simulink model "MesurementModel"  (R2023b)
settings: configuration reference "Configuration" (kept outside this file)
libraries: dspstat3 x4, SignalEditorBlockLib x1
settings Model: DataDictionary=ZC_EVPowerSystem.sldd  Creator=ykamatan  LastModifiedBy=ykamatan
settings ConfigSetRef: SourceName=Configuration

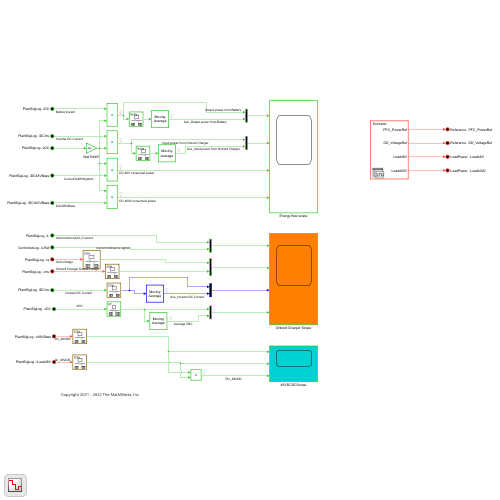
[thumbnail: Simulink's stored preview of the top-level diagram]
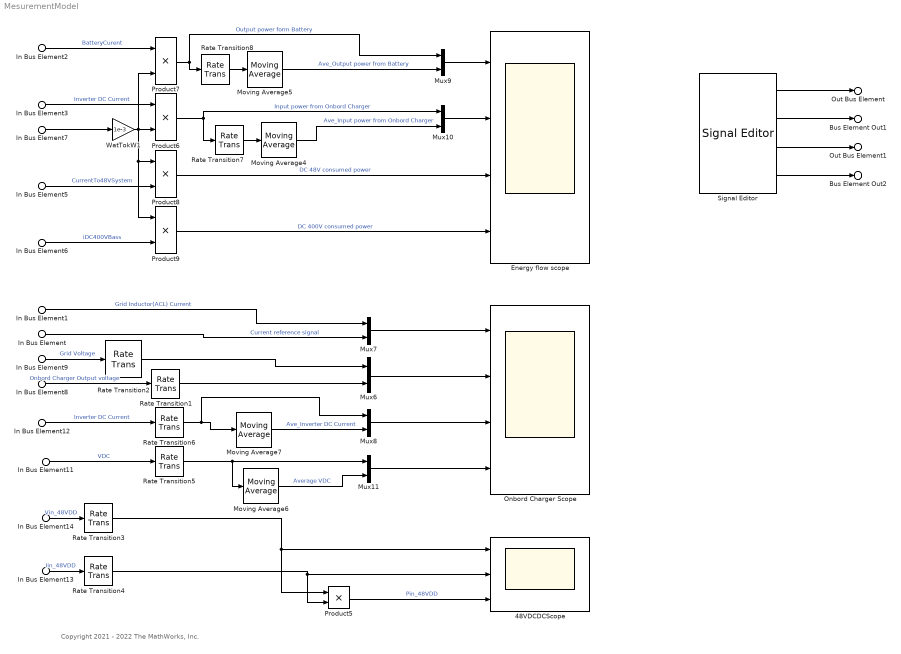
== system MesurementModel ==
  note: Copyright 2021 - 2022 The MathWorks, Inc.
  In Bus Element1 : Inport  PortName=PlantSigLog  Element=iL
  In Bus Element2 : Inport  PortName=PlantSigLog  Element=iDC
  In Bus Element3 : Inport  PortName=PlantSigLog  Element=iDCInv
  In Bus Element12 : Inport  PortName=PlantSigLog  Element=iDCInv
  In Bus Element13 : Inport  PortName=PlantSigLog  Element=iLoad48V
  In Bus Element5 : Inport  PortName=PlantSigLog  Element=iDC48VBass
  In Bus Element6 : Inport  PortName=PlantSigLog  Element=iDC400VBass
  In Bus Element7 : Inport  PortName=PlantSigLog  Element=vDC
  In Bus Element11 : Inport  PortName=PlantSigLog  Element=vDC
  In Bus Element8 : Inport  PortName=PlantSigLog  Element=vInv
  In Bus Element9 : Inport  PortName=PlantSigLog  Element=vs
  In Bus Element14 : Inport  PortName=PlantSigLog  Element=v48VBass
  In Bus Element : Inport  Port=2  PortName=ControllerLog  Element=iLRef
  48VDCDCScope : Scope  NumInputPorts=3
  Energy flow scope : Scope  NumInputPorts=4
  Moving Average{4..7} (4 alike) : dspstat3/Moving Average  Method=Sliding window  ForgettingFactorPort=off  SpecifyWindowLength=on  WindowLength=1000  OverlapLength=999  AllowArbitraryInputLength=off  ForgettingFactor=0.9  SimulateUsing=Code generation
  Mux{6..11} (6 alike) : Mux  Inputs=2
  Onbord Charger Scope : Scope  NumInputPorts=4
  Product{5..9} (5 alike) : Product
  Rate Transition{1..5,7..8} (7 alike) : RateTransition  OutPortSampleTime=1/1000
  Rate Transition6 : RateTransition  OutPortSampleTime=1/100
  Signal Editor : SignalEditorBlockLib/Signal Editor  FileName=InputSignal.mat  ActiveScenario=Scenario  ActiveSignal=DD_VoltageRef  IsBus=off  OutputBusObjectStr=Bus: BusObject  SampleTime=1/10000  ZeroCross=off  OutputAfterFinalValue=Setting to zero  Unit=inherit  PreserveSignalName=on  ApplySigPropsToAllScenarios=on  ApplySigPropsToAllSignals=off
  WatTokW1 : Gain  Gain=1e-3
  Out Bus Element : Outport  PortName=Reference  Element=PFC_PowerRef
  Bus Element Out1 : Outport  PortName=Reference  Element=DD_VoltageRef
  Out Bus Element1 : Outport  Port=2  PortName=LoadPower  Element=Load48V
  Bus Element Out2 : Outport  Port=2  PortName=LoadPower  Element=Load400V
  wires:
  Signal Editor/1 -> Out Bus Element/1
  Signal Editor/2 -> Bus Element Out1/1
  Signal Editor/3 -> Out Bus Element1/1
  Signal Editor/4 -> Bus Element Out2/1
  Product8/1 -> Energy flow scope/3  "DC 48V consumed power"
  Product9/1 -> Energy flow scope/4  "DC 400V consumed power"
  Mux10/1 -> Energy flow scope/2
  Moving Average6/1 -> Mux11/2  "Average VDC"
  In Bus Element6/1 -> Product9/2  "iDC400VBass"
  WatTokW1/1 -> Product9/1, Product8/1, Product6/2, Product7/2
  In Bus Element3/1 -> Product6/1  "Inverter DC Current"
  In Bus Element5/1 -> Product8/2  "CurrentTo48VSystem"
  In Bus Element1/1 -> Mux7/1  "Grid Inductor(ACL) Current"
  In Bus Element9/1 -> Rate Transition2/1  "Grid Voltage"
  In Bus Element14/1 -> Rate Transition3/1  "Vin_48VDD"
  In Bus Element11/1 -> Rate Transition5/1  "VDC"
  Moving Average7/1 -> Mux8/2  "Ave_Inverter DC Current"
  Product7/1 -> Mux9/1, Rate Transition8/1  "Output power form Battery"
  In Bus Element12/1 -> Rate Transition6/1  "Inverter DC Current"
  In Bus Element13/1 -> Rate Transition4/1  "Iin_48VDD"
  Product6/1 -> Rate Transition7/1, Mux10/1  "Input power from Onbord Charger"
  Mux9/1 -> Energy flow scope/1
  In Bus Element8/1 -> Rate Transition1/1  "Onbord Charger Output voltage"
  Moving Average4/1 -> Mux10/2  "Ave_Input power from Onbord Charger"
  In Bus Element/1 -> Mux7/2  "Current reference signal"
  Mux7/1 -> Onbord Charger Scope/1
  Mux11/1 -> Onbord Charger Scope/4
  Mux6/1 -> Onbord Charger Scope/2
  In Bus Element2/1 -> Product7/1  "BatteryCurent"
  Product5/1 -> 48VDCDCScope/3  "Pin_48VDD"
  Mux8/1 -> Onbord Charger Scope/3
  Moving Average5/1 -> Mux9/2  "Ave_Output power from Battery"
  In Bus Element7/1 -> WatTokW1/1
  Rate Transition5/1 -> Moving Average6/1, Mux11/1
  Rate Transition6/1 -> Mux8/1, Moving Average7/1
  Rate Transition7/1 -> Moving Average4/1
  Rate Transition8/1 -> Moving Average5/1
  Rate Transition1/1 -> Mux6/2
  Rate Transition2/1 -> Mux6/1
  Rate Transition3/1 -> Product5/1, 48VDCDCScope/1
  Rate Transition4/1 -> 48VDCDCScope/2, Product5/2
